simulink model "PID_Algorithm"  (R2024b)
settings: Solver=VariableStepAuto  StartTime=0.0  StopTime=10.0  RelTol=1e-3
settings Model: Creator=fawaz  LastModifiedBy=fawaz

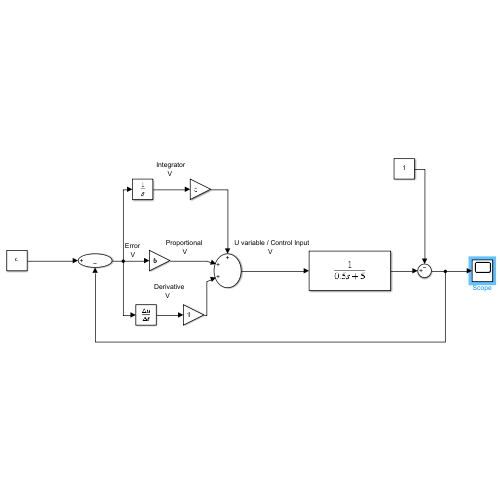
[thumbnail: Simulink's stored preview of the top-level diagram]
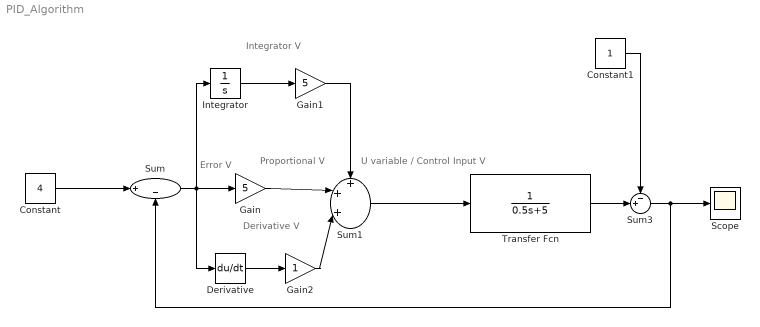
== system PID_Algorithm ==
  note: Derivative
      |       V
  note: Integrator
      |       V
  note: Error
      |    V
  note: U variable / Control Input
      |                   V
  note: Proportional
      |          V
  Constant : Constant  Value=4
  Constant1 : Constant
  Derivative : Derivative
  Gain : Gain  Gain=5
  Gain1 : Gain  Gain=5
  Gain2 : Gain
  Integrator : Integrator
  Scope : Scope
  Sum : Sum  Inputs=|+-
  Sum1 : Sum  Inputs=+++|
  Sum3 : Sum  Inputs=-+|
  Transfer Fcn : TransferFcn  Denominator=[0.5 5]
  wires:
  Constant/1 -> Sum/1
  Sum/1 -> Derivative/1, Integrator/1, Gain/1
  Sum1/1 -> Transfer Fcn/1
  Gain/1 -> Sum1/2
  Integrator/1 -> Gain1/1
  Gain1/1 -> Sum1/1
  Gain2/1 -> Sum1/3
  Derivative/1 -> Gain2/1
  Constant1/1 -> Sum3/1
  Transfer Fcn/1 -> Sum3/2
  Sum3/1 -> Scope/1, Sum/2
